simulink model "LAB6T3_v3"  (R2018b)
settings: Solver=VariableStepAuto  StartTime=0.0  StopTime=100  RelTol=1e-3
libraries: aerolibanim x1
settings Model: Creator=aloisia  LastModifiedBy=aloisia

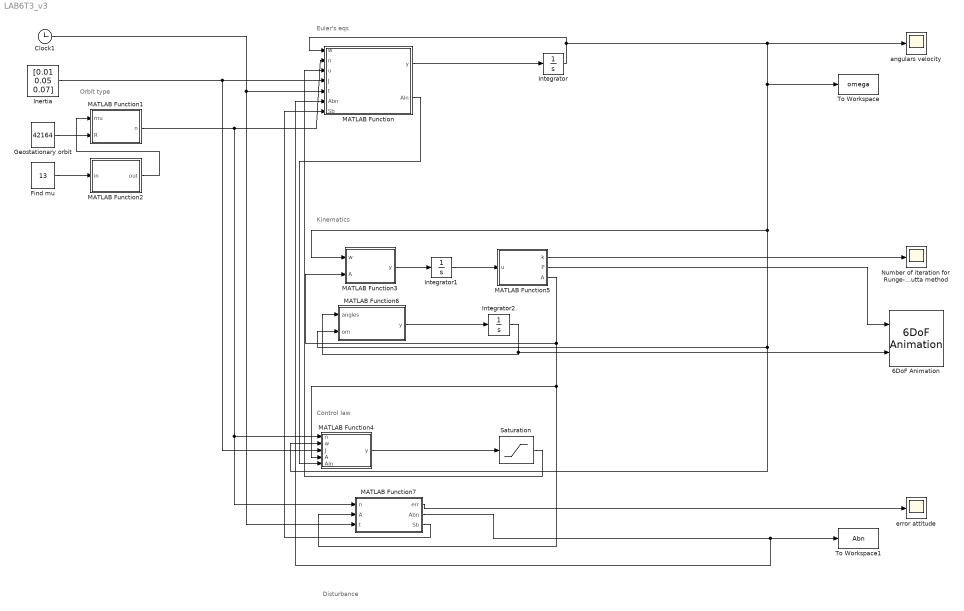
== system LAB6T3_v3 ==
  note: Orbit type
  note: Disturbance
  note: Control law
  note: Kinematics
  note: Euler's eqs
  6DoF Animation : aerolibanim/6DoF Animation  u1=[0 4000 -2000 2000 -5000 -3000]  u2=0.07  u3=800  u4=[4000 0 -5000]  u5=Fixed position  u6=[2000 500 -3150]  u7=10  u8=on
      settings: SourceProductName=Aerospace Blockset
  Clock1 : Clock
  Find mu : Constant  Tag=J  Description=J  Value=13
  Geostationary orbit : Constant  Tag=J  Description=J  Value=42164
  "Inertia " : Constant  Tag=J  Description=J  Value=[0.01 0.05 0.07]
  Integrator : Integrator  InitialCondition=[0.01;0.01;0.03]
  Integrator1 : Integrator  InitialCondition=[-0.782 0 -0.6233; 0.6233 0 -0.782; 0 -1 0]
  Integrator2 : Integrator  InitialCondition=[0;0;0]
  MATLAB Function : MATLAB Function  TreatAsAtomicUnit=on
  MATLAB Function1 : MATLAB Function  TreatAsAtomicUnit=on
  MATLAB Function2 : MATLAB Function  TreatAsAtomicUnit=on
  MATLAB Function3 : MATLAB Function  TreatAsAtomicUnit=on
  MATLAB Function4 : MATLAB Function  TreatAsAtomicUnit=on
  MATLAB Function5 : MATLAB Function  TreatAsAtomicUnit=on
  MATLAB Function6 : MATLAB Function  TreatAsAtomicUnit=on
  MATLAB Function7 : MATLAB Function  TreatAsAtomicUnit=on
  Number of iteration for Runge-Kutta method : Scope
  Saturation : Saturate  UpperLimit=0.01  LowerLimit=-0.1  LinearizeAsGain=off  ZeroCross=off
  To Workspace : ToWorkspace  VariableName=omega  SampleTime=-1
  To Workspace1 : ToWorkspace  VariableName=Abn  SampleTime=-1
  "angulars velocity " : Scope
  error attitude : Scope
  wires:
  MATLAB Function/1(y) -> Integrator/1
  Find mu/1 -> MATLAB Function2/1(in)
  Geostationary orbit/1 -> MATLAB Function1/2(R)
  MATLAB Function2/1(out) -> MATLAB Function1/1(mu)
  MATLAB Function4/1(y) -> Saturation/1
  Saturation/1 -> MATLAB Function/3(u)
  MATLAB Function3/1(y) -> Integrator1/1
  Integrator1/1 -> MATLAB Function5/1(u)
  MATLAB Function5/3(A) -> MATLAB Function4/4(A), MATLAB Function7/2(A), MATLAB Function3/2(A)
  MATLAB Function5/1(k) -> Number of iteration for Runge-Kutta method/1
  MATLAB Function5/2(P) -> 6DoF Animation/1
  Integrator2/1 -> MATLAB Function6/1(angles), 6DoF Animation/2
  MATLAB Function6/1(y) -> Integrator2/1
  Integrator/1 -> MATLAB Function/1(w), MATLAB Function6/2(om), MATLAB Function4/2(w), MATLAB Function3/1(w), To Workspace/1, "angulars velocity "/1
  MATLAB Function/2(Aln) -> MATLAB Function4/5(Aln)
  MATLAB Function1/1(n) -> MATLAB Function4/1(n), MATLAB Function7/1(n), MATLAB Function/2(n)
  "Inertia "/1 -> MATLAB Function/4(J), MATLAB Function4/3(J)
  MATLAB Function7/1(err) -> error attitude/1
  MATLAB Function7/2(Abn) -> MATLAB Function/6(Abn), To Workspace1/1
  MATLAB Function7/3(Sb) -> MATLAB Function/7(Sb)
  Clock1/1 -> MATLAB Function7/3(t), MATLAB Function/5(t)

== matlab function LAB6T3_v3/MATLAB Function1 ==
  data: mu input; n output; R input
function n = circular(mu,R)

% This function provides to calculate the angular velocity of a circular
% orbit

 R=42168;
 n=(mu/(R^3))^0.5 ;
end

== matlab function LAB6T3_v3/MATLAB Function ==
  data: w input; n input; u input; y output; J input; t input; Abn input; Aln output; Sb input
function [y,Aln] = euler(w, n,u,J,t,Abn,Sb)

%Set Data

Ix=J(1); Iy=J(2); Iz=J(3) ;
wx=w(1) ; wy=w(2); wz=w(3);
wdot=zeros(3,1);

%Gravity Gradiant

Aln = [cos(n*t) sin(n*t) 0 ; -sin(n*t) cos(n*t) 0; 0 0 1];
Abl = Abn*(Aln');
c = Abl*[1;0;0];
Ma1 = (3*(n^2))*((Iz-Iy)*c(3)*c(2)) ;
Ma2 = (3*(n^2))*((Ix-Iz)*c(1)*c(3)) ;
Ma3 = (3*(n^2))*((Iy-Ix)*c(1)*c(2));

% SRP disturbance

n1=[1;0;0]; n4=-n1;
n2=[0;1;0]; n5=-n2;
n3=[0;0;1]; n6=-n3;

N =[n1 n2 n3 n4 n5 n6];

a=0.50;                 %[m]                                    
A = a*2;                %[m^2]
P = 1358/(300000*1e3);  %[W/m^2]/[m/s]
rho_s=0.5;              %[kg/m^3]
rho_d=0.1;              %[kg/m^3]
F = zeros(3,6);         %[N]
br = 0.1*a*N;           %[m] arm is usually 10% of the total dimension
M=zeros(3,6);


for i = 1:6
    
    if dot(Sb,N(:,i))>0
        F(:,i)= P*A * dot(Sb,N(:,i)) * ((1-rho_s)*Sb + (2*rho_s *dot(Sb,N(:,i))...
            + 2/3 * rho_d)* N(:,i));
    else
        F(:,i) = zeros(3,1);
     
    end
  M(:,i)=cross(F(:,i),br(:,i));  
end

M=M';
Mt=sum(M(:,1:3));



%% Euler Equation
wdot(1)= ((Iy-Iz)/Ix)*wy*wz+u(1)/Ix+Ma1/Ix+Mt(1)/Ix;
wdot(2)= ((Iz-Ix)/Iy)*wx*wz+u(2)/Iy+Ma2/Iy+Mt(2)/Iy;
wdot(3)= ((Ix-Iy)/Iz)*wx*wy+u(3)/Iz+Ma3/Iz+Mt(3)/Iz;


y = wdot;
Aln = Aln;
end

== matlab function LAB6T3_v3/MATLAB Function2 ==
  data: in input; out output

function out = astroConstants(in)
coder.extrinsic('warning')
% astroConstants.m - Returns astrodynamic-related physical constants.
%
% PROTOTYPE:
%   out = astro_constants(in)
%
% DESCRIPTION:
%   Returns a row vector of constants, in which there is the corresponding
%   constant for each element of the input vector.
%
%   List of identifiers:
%       Generic astronomical constants:
%           1   Universal gravity constant (G) (from DITAN) [km^3/(kg*s^2)]
%           2   Astronomical Unit (AU) (from DITAN) [km]
%       Sun related:
%           3   Sun mean radius (from DITAN) [km]
%           4   Sun planetary constant (mu = mass * G) (from DITAN)
%               [km^3/s^2]
%           31  Energy flux density of the Sun (from Wertz,SMAD)
%               [W/m2 at 1 AU]
%       Other:
%           5   Speed of light in the vacuum (definition in the SI) [km/s]
%           6   Standard free fall (the acceleration due to gravity on the
%               Earth's surface at sea level) (from Wertz,SMAD) [m/s^2]
%           7   Mean distance Earth-Moon (from Wertz,SMAD) [km]
%           8   Obliquity (angle) of the ecliptic at Epoch 2000 (from
%               Wertz,SMAD) [rad]
%           9   Gravitatonal field constant of the Earth (from Wertz,SMAD,
%               taken from JGM-2). This should be used in conjunction to
%               Earth radius = 6378.1363 km 
%       Planetary constants of the planets (mu = mass * G) [km^3/s^2]:
%           11  Me      (from DITAN)
%           12  V       (from DITAN)
%           13  E       (from DITAN)
%           14  Ma      (from DITAN)
%           15  J       (from DITAN)
%           16  S       (from DITAN)
%           17  U       (from DITAN)
%           18  N       (from DITAN)
%           19  P       (from DITAN)
%           20  Moon    (from DITAN)
%       Mean radius of the planets [km]:
%           21  Me      (from DITAN)
%           22  V       (from DITAN)
%           23  E       (from DITAN)
%           24  Ma      (from DITAN)
%           25  J       (from DITAN)
%           26  S       (from DITAN)
%           27  U       (from DITAN)
%           28  N       (from DITAN)
%           29  P       (from DITAN)
%           30  Moon    (from DITAN)
%
%   Notes for upgrading this function:
%       It is possible to add new constants.
%       - DO NOT change the structure of the function, as well as its
%           prototype.
%       - DO NOT change the identifiers of the constants that have already
%           been defined in this function. If you want to add a new
%           constant, use an unused identifier.
%       - DO NOT add constants that can be easily computed starting form
%           other ones (avoid redundancy).
%       Contact the author for modifications.
%
% INPUT:
%   in      Vector of identifiers of required constants.
%
% OUTPUT:
%   out     Vector of constants.
%
% EXAMPLE:
%   astroConstants([2, 4, 26])
%      Returns a row vector in which there is the value of the AU, the Sun
%      planetary constant and the mean radius of Saturn.
%
%   astroConstants(10 + [1:9])
%      Returns a row vector with the planetary constant of each planet.
%
% REFERENCES:
%   - DITAN (Direct Interplanetary Trajectory Analysis), Massimiliano
%       Vasile, 2006.
%	- Wertz J. R., Larson W. J., "Space Mission Analysis and Design", Third
%       Edition, Space Technology Library 2003.
%
% CALLED FUNCTIONS:
%   (none)
%
% AUTHOR:
%   Matteo Ceriotti, 2006, MATLAB, astroConstants.m
%
% PREVIOUS VERSION:
%   Matteo Ceriotti, 2006, MATLAB, astro_constants.m, Ver. 1.2
%       - Header and function name in accordance with guidlines.
%
% CHANGELOG:
%   26/10/2006, Camilla Colombo: Updated.
%   22/10/2007, Camilla Colombo: astroConstants(8) added (Obliquity (angle)
%       of the ecliptic at Epoch 2000).
%   02/10/2009, Camilla Colombo: Header and function name in accordance
%       with guidlines.
%   12/11/2010, Camilla Colombo: astroConstants(9) added (J2) Note: the
%       present value of J2 is not consistent with the value of the Earth
%       radius. This value of J2 should be used in conjunction to Earth
%       radius = 6378.1363 km 
%
% -------------------------------------------------------------------------
% LAST UPDATE : adapted version for R2018b Simulink version from Aloisia Russo for the
%               Spacecraft Attitude Dynamics and Control course. 

out = zeros(length(in));
for i=1:length(in)
   
    switch in(i)
        case 1
            out(i)=6.67259e-20; % From DITAN
        case 2
            out(i)=149597870.7; % From DITAN
        case 3
            out(i)=700000; % From DITAN
        case 4
            %out(i)=0.19891000000000E+31*6.67259e-20; % From DITAN
            out(i)=1.988919445342813e+030*6.67259e-20; % From NASA
        case 5
            out(i)=299792.458; % Definition in the SI
        case 6
            out(i)=9.80665; % Definition in Wertz, SMAD
        case 7
            out(i)=384401; % Definition in Wertz, SMAD
        case 8
            out(i)=23.43928111*pi/180; % Definition in Wertz, SMAD
        case 9
            out(i)=0.1082626925638815e-2; % Definition in Wertz, SMAD
        case 11
            out(i)=0.33020000000000E+24*6.67259e-20; % From DITAN
        case 12
            out(i)=0.48685000000000E+25*6.67259e-20; % From DITAN
        case 13
            out(i)=0.59736990612667E+25*6.67259e-20; % From DITAN
        case 14
            out(i)=0.64184999247389E+24*6.67259e-20; % From DITAN
        case 15
            out(i)=0.18986000000000E+28*6.67259e-20; % From DITAN
        case 16
            out(i)=0.56846000000000E+27*6.67259e-20; % From DITAN
        case 17
            out(i)=0.86832000000000E+26*6.67259e-20; % From DITAN
        case 18
            out(i)=0.10243000000000E+27*6.67259e-20; % From DITAN
        case 19
            out(i)=0.14120000000000E+23*6.67259e-20; % From DITAN
        case 20
            out(i)=0.73476418263373E+23*6.67259e-20; % From DITAN
        case 21
            out(i)=0.24400000000000E+04; % From DITAN
        case 22
            out(i)=0.60518000000000E+04; % From DITAN
        case 23
            out(i)=0.63781600000000E+04; % From DITAN
        case 24
            out(i)=0.33899200000000E+04; % From DITAN
        case 25
            out(i)=0.69911000000000E+05; % From DITAN
        case 26
            out(i)=0.58232000000000E+05; % From DITAN
        case 27
            out(i)=0.25362000000000E+05; % From DITAN
        case 28
            out(i)=0.24624000000000E+05; % From DITAN
        case 29
            out(i)=0.11510000000000E+04; % From DITAN
        case 30
            out(i)=0.17380000000000E+04; % From DITAN
        case 31
            out(i)=1367; % From Wertz, SMAD
        % Add an identifier and constant here. Prototype:
        % case $identifier$
        %     out(i)=$constant_value$;
        otherwise
            warning('Constant identifier %d is not defined!',in(i));
            out(i)=0;
    end
end

== matlab function LAB6T3_v3/MATLAB Function3 ==
  data: w input; y output; A input
function y = kinematics(w,A)


W=[0 -w(3) w(2); w(3) 0 -w(1); -w(2) -w(1) 0];

Adot=-W*A ;

y=Adot ;
end

== matlab function LAB6T3_v3/MATLAB Function4 ==
  data: n input; w input; y output; J input; A input; Aln input
function y  = control(n,w,J,A,Aln)

%Function to perform the control: note that circular orbits are considered

% Set gain
k1=0.5; k2=0.5;

% Control law 
Jd=diag(J); 
K1=k1*Jd ; K2=k2*Jd;
Ad=Aln;
%Ad = eye(3);
Ae=A*Ad' ;
Q=(Ae')-Ae ;
e=[Q(3,2) Q(1,3) Q(2,1)]';


 wln = [0;0;n];
 we = w - Ae*wln;
 
u=-K1*we-K2*e;

y=u;

end

== matlab function LAB6T3_v3/MATLAB Function5 ==
  data: k output; P output; u input; A output
function [k,P,A]  = ortho(u)

c=1; A=u; k=0;
while c>0.000001

A=(1.5.*A)-(A*(A')*A./2) ; % Runge-Kutta method
c=trace((eye(3)-(A')*A)) ; % error
k=k+1 ; %counter
end

z=k;
P = A * [1;0;0];

end

== matlab function LAB6T3_v3/MATLAB Function6 ==
  data: angles input; y output; om input
function y = small_angle_kin(angles,om)

% This function provides the calculation of A by using 
% Phi, theta, psi and omega in Radiants
phi = angles(1);
theta = angles(2);
psi = angles(3);

phidot = (om(1)*cos(psi) - om(2)*sin(psi)) / cos(theta);
thetadot = om(2)*cos(psi) + om(1)*sin(psi);
psidot = om(3) - (om(1)*cos(psi) - om(2)*sin(psi))* sin(theta)/cos(theta);
anglesdot = [phidot; thetadot; psidot];

y = anglesdot;
end

== matlab function LAB6T3_v3/MATLAB Function7 ==
  data: n input; A input; err output; t input; Abn output; Sb output
function [err,Abn,Sb] = TRIAD(n,A,t)

    %LAB 6: TASK 3
    %Circular orbit is considered
    
    n = n;                          % Mean motion
    B = pi/6 + 150*n;               % Initial phase (150s from previous detumbling)
    ep = 23.45*pi/180;              % Ecliptic inclination
    
    % Sun pointing vector
    Sn = [cos(n*t+B); sin(n*t+B)*cos(ep); sin(n*t+B)*sin(ep)];
    Sb = A*Sn;                      % Model of the sensor behaviour
    
    % Earth horizon pointing vector
    
    hn = -[cos(n*t) sin(n*t) 0]';
    hb = A*hn;                      % Model of the sensor behaviour
    
    %Accuracy error
    
    es = 1/60 * pi/180;
    ee = 6/60 * pi/180;
    Aes = [cos(es)*cos(es) cos(es)*sin(es)*sin(es)+sin(es)*cos(es) -cos(es)*sin(es)*cos(es)+sin(es)*sin(es);...
          -sin(es)*cos(es) -sin(es)*sin(es)*sin(es)+cos(es)*cos(es) sin(es)*sin(es)*cos(es)+cos(es)*sin(es);...
          sin(es) -cos(es)*sin(es) cos(es)*cos(es)];
      
    Aee = [cos(ee)*cos(ee) cos(ee)*sin(ee)*sin(ee)+sin(ee)*cos(ee) -cos(ee)*sin(ee)*cos(ee)+sin(ee)*sin(ee);...
      -sin(ee)*cos(ee) -sin(ee)*sin(ee)*sin(ee)+cos(ee)*cos(ee) sin(ee)*sin(ee)*cos(ee)+cos(ee)*sin(ee);...
      sin(ee) -cos(ee)*sin(ee) cos(ee)*cos(ee)];
  
    %Sensors data considering the accuracy
    
    hb = Aee *hb/norm(hb);
    hb_noerr = hb/norm(hb);
    Sb = Aes * Sb/norm(Sb);
    Sb_noerr =  Sb/norm(Sb);
    

    SbXhb = cross(Sb,hb);
    SnXhn = cross(Sn,hn);
    Vb = [ Sb  SbXhb/norm(SbXhb) cross(Sb,SbXhb/norm(SbXhb))]; 
    Vn = [ Sn  SnXhn/norm(SnXhn) cross(Sn,SnXhn/norm(SnXhn))]; 
    Abn = Vb*Vn';
    
   %err = (A - Abn);
   err = abs(norm(Sb - Abn*Sn));
   
end
